simulink model "mppt_fractional_fuzzy_v1"  (R2019a)
settings: Solver=FixedStepAuto  StartTime=0.0  StopTime=3  FixedStep=1e-6  RelTol=1e-3
undefined symbols (not defined in the file): sigbuilder_block, Tpwm
libraries: powerlib x8, fuzblock x1, re_lib x1, eePwmGenerator x1
settings Model: Creator=asus  LastModifiedBy=asus

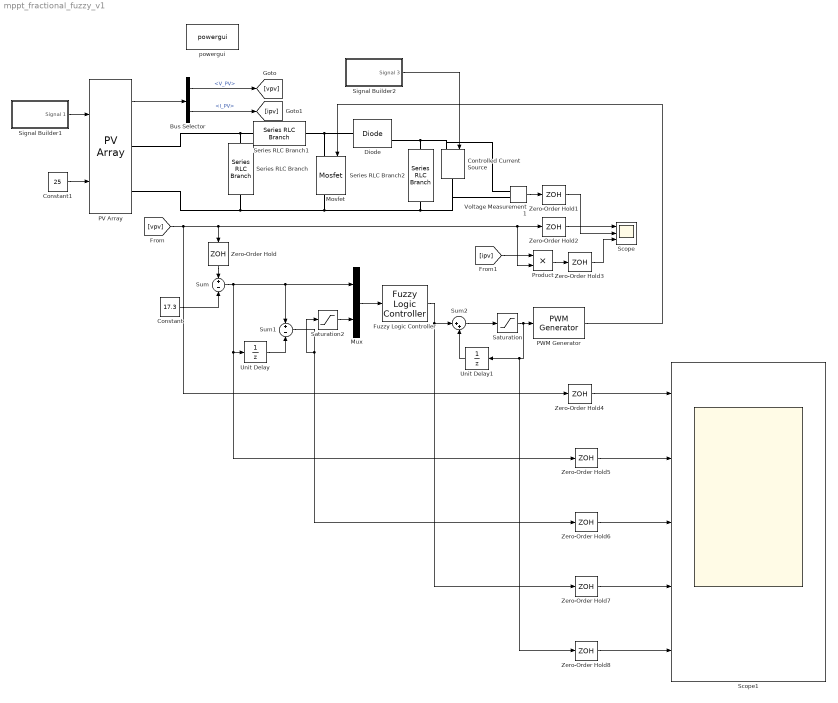
== system mppt_fractional_fuzzy_v1 ==
  Bus Selector : BusSelector  OutputSignals=V_PV,I_PV
  Constant : Constant  Value=17.3
  Constant1 : Constant  Value=25
  Controlled Current Source : powerlib/Electrical Sources/Controlled Current Source  Initialize=on  Source_Type=AC  Amplitude=0  Phase=0  Frequency=0  Measurements=None
      settings: SourceProductName=Simscape Electrical
  Diode : powerlib/Power Electronics/Diode  Ron=0.001  Lon=0  Vf=0.8  IC=0  UseSnubber=0  Rs=500  Cs=250e-9  Measurements=on
      settings: SourceProductName=Simscape Electrical
  Fuzzy Logic Controller : fuzblock/Fuzzy Logic  Controller  FIS=mppt_fractional  OutputSampleNumber=101  DataType=double  FuzzifiedInputs=off  RuleFiringStrengths=off  RuleOutputs=off  AggregatedOutputs=off  SimulateUsing=Interpreted execution  OutOfRangeInputValueMessage=warning  NoRuleFiredMessage=warning  EmptyOutputFuzzySetMessage=warning
  Mosfet : powerlib/Power Electronics/Mosfet  Ron=0.1  Lon=0  Rd=0.01  Vfd=0  IC=0  Rs=1e5  Cs=inf  Measurements=on
      settings: SourceProductName=Simscape Electrical
  Mux : Mux  Inputs=2
  PV Array : re_lib/Solar/PV Array  Npar=1  Nser=1  PlotType=array @ 1000 W/m2 & specified temperatures  S_vec="[ 1000  500  100 ]"  Temp_C_vec="[ 45 25  ]"  ModuleName=Apollo Solar Energy ASEC-120G6M  PlotWhenSelected=off  Pm=120.0969  Ncell=36  Voc=21.6  Isc=7.49  Vm=17.33  Im=6.93  beta_Voc_pc=-0.32991  alpha_Isc_pc=0.021402  beta_Voc=-0.07126  alpha_Isc=0.001603  IL=7.5105  I0=7.9614e-11  nI=0.92533  Rsh=90.7546  Rs=0.24853  BAL=off  Tc=1e-6  Tfilter=5e-5
      settings: SourceProductName=Simscape Electrical
  PWM Generator : eePwmGenerator/PWM Generator  CarrCount=Up  Tper=Tpwm  Ts=1e-6
      settings: SourceProductName=Simscape Electrical
  Product : Product
  Saturation : Saturate  UpperLimit=.98  LowerLimit=.01
  Saturation2 : Saturate  UpperLimit=2.5  LowerLimit=-2.5
  Scope : Scope  NumInputPorts=3
  Scope1 : Scope  NumInputPorts=5
  Series RLC Branch : powerlib/Elements/Series RLC Branch  LConnTagsString=__new0  RConnTagsString=__new0  BranchType=C  Resistance=1  Inductance=1e-3  SetiL0=off  InitialCurrent=0  Capacitance=10e-6  Setx0=off  InitialVoltage=0  Measurements=None
      settings: SourceProductName=Simscape Electrical
  Series RLC Branch1 : powerlib/Elements/Series RLC Branch  LConnTagsString=__new0  RConnTagsString=__new0  BranchType=L  Resistance=1  Inductance=1e-3  SetiL0=off  InitialCurrent=0  Capacitance=10e-6  Setx0=off  InitialVoltage=0  Measurements=None
      settings: SourceProductName=Simscape Electrical
  Series RLC Branch2 : powerlib/Elements/Series RLC Branch  LConnTagsString=__new0  RConnTagsString=__new0  BranchType=C  Resistance=1  Inductance=1e-3  SetiL0=off  InitialCurrent=0  Capacitance=2000e-6  Setx0=off  InitialVoltage=0  Measurements=None
      settings: SourceProductName=Simscape Electrical
  Signal Builder1 : Subsystem  Tag=STV Subsys  LoadFcn=sigbuilder_block('load',[83.5 110.5 550.5 362.5 ]);  StartFcn=sigbuilder_block('start');  StopFcn=sigbuilder_block('stop');  ClipboardFcn=sigbuilder_block('clipboard');  mask(Sigbuilder block){tuvar=[0:10]}
      mask help: Simulink:masks:SigbuilderBlock_MD
      mask init:
      | if ~strcmp(get_param(bdroot(gcbh),'SimulationStatus'),'stopped') tuvar = sigbuilder_block('maskInit'); end
      settings: CopyFcn=sigbuilder_block('copy');  DeleteFcn=sigbuilder_block('delete');  ModelCloseFcn=sigbuilder_block('modelClose');  PreSaveFcn=sigbuilder_block('preSave');  PauseFcn=sigbuilder_block('pause');  ContinueFcn=sigbuilder_block('continue');  NameChangeFcn=sigbuilder_block('namechange');  OpenFcn=sigbuilder_block('open',[83.5 110.5 550.5 362.5 ]);  CloseFcn=sigbuilder_block('close');
      mask Display: plot(0, 0, 100, 100,[2, 2, 32, 32, 2], [68, 8, 8, 68, 68],[32, 2], [38, 38], [32, 19, 2],[53, 60, 44], [32, 17, 17, 2],[16, 16, 31, 31]);txt = getActiveGroup(gcbh);text(2, 100, txt,'verticalAlignment', 'top');
  Signal Builder2 : Subsystem  Tag=STV Subsys  LoadFcn=sigbuilder_block('load',[0 30 960 455.5 ]);  StartFcn=sigbuilder_block('start');  StopFcn=sigbuilder_block('stop');  ClipboardFcn=sigbuilder_block('clipboard');  mask(Sigbuilder block){tuvar=[0:10]}
      mask help: Simulink:masks:SigbuilderBlock_MD
      mask init:
      | if ~strcmp(get_param(bdroot(gcbh),'SimulationStatus'),'stopped') tuvar = sigbuilder_block('maskInit'); end
      settings: CopyFcn=sigbuilder_block('copy');  DeleteFcn=sigbuilder_block('delete');  ModelCloseFcn=sigbuilder_block('modelClose');  PreSaveFcn=sigbuilder_block('preSave');  PauseFcn=sigbuilder_block('pause');  ContinueFcn=sigbuilder_block('continue');  NameChangeFcn=sigbuilder_block('namechange');  OpenFcn=sigbuilder_block('open',[5.5 30 949 418 ]);  CloseFcn=sigbuilder_block('close');
      mask Display: plot(0, 0, 100, 100,[2, 2, 32, 32, 2], [68, 8, 8, 68, 68],[32, 2], [38, 38], [32, 19, 2],[53, 60, 44], [32, 17, 17, 2],[16, 16, 31, 31]);txt = getActiveGroup(gcbh);text(2, 100, txt,'verticalAlignment', 'top');
  Sum : Sum  Inputs=+-
  Sum1 : Sum  Inputs=+-
  Sum2 : Sum  Inputs=|++
  Unit Delay : UnitDelay  SampleTime=-1  HasFrameUpgradeWarning=on
  Unit Delay1 : UnitDelay  SampleTime=-1  HasFrameUpgradeWarning=on
  Voltage Measurement1 : powerlib/Measurements/Voltage Measurement  PhasorSimulation=off  OutputType=Complex  PSBequivalent=0
      settings: SourceProductName=Simscape Electrical
  Zero-Order Hold{,1..8} (9 alike) : ZeroOrderHold  SampleTime=5*Tpwm
  powergui : powerlib/powergui  Priority=1  SimulationMode=Discrete  SampleTime=1e-6  frequency=60  Iterations=50  frequencyindice=0  Pbase=100e6  ErrMax=1e-4  UnitsV=kV  UnitsW=MW  buscounter=0  FunctionMessages=off  echomessages=off  EnableUseOfTLC=off  CurrentSourceSwitches=off  DisableSnubberDevices=off  DisableRonSwitches=off  DisableVfSwitches=off  DisplayEquations=off  AutomaticDiscreteSolvers=off  SolverType=Tustin/Backward Euler (TBE)  Interpol=off  ExternalGateDelay=off  methode=off  Ts=100  x0status=blocks  SPID=on  SwTol=0  HookPort=off  NonlinearTolerance=0  nMaxIteration=15  ContinueOnMaxIteration=off  RestoreLinks=warning  ResistiveCurrentMeasurement=off  Frange=[0:2:500]  Ylog=off  Xlog=on  ShowGrid=off  save=off  variable=ZData  structure=0  ZoomFFT=off  StartTime=0.0  cycles=1  DisplayStyle=1  fundamental=60  FreqAxis=off  MaxFrequency=1000  frequencyindicesteady=1  RmsSteady=1  display=off
      settings: SourceProductName=Simscape Electrical
  wires:
  Signal Builder1/1(Signal 1) -> PV Array/1
  Constant1/1 -> PV Array/2
  Constant/1 -> Sum/2
  Sum2/1 -> Saturation/1
  PWM Generator/1 -> Mosfet/1
  Zero-Order Hold/1 -> Sum/1
  [vpv] -> Zero-Order Hold4/1, Zero-Order Hold/1, Zero-Order Hold2/1, Product/2
  Signal Builder2/1(Signal 3) -> Controlled Current Source/1
  Voltage Measurement1/1 -> Zero-Order Hold1/1
  [ipv] -> Product/1
  Saturation/1 -> Zero-Order Hold8/1, Unit Delay1/1, PWM Generator/1
  PV Array/1 -> Bus Selector/1
  Bus Selector/1 -> [vpv]  "<V_PV>"
  Bus Selector/2 -> [ipv]  "<I_PV>"
  Unit Delay/1 -> Sum1/2
  Sum1/1 -> Saturation2/1, Zero-Order Hold6/1
  Mux/1 -> Fuzzy Logic Controller/1
  Fuzzy Logic Controller/1 -> Zero-Order Hold7/1, Sum2/1
  Unit Delay1/1 -> Sum2/2
  Sum/1 -> Sum1/1, Mux/1, Zero-Order Hold5/1, Unit Delay/1
  Saturation2/1 -> Mux/2
  Zero-Order Hold1/1 -> Scope/2
  Zero-Order Hold2/1 -> Scope/1
  Product/1 -> Zero-Order Hold3/1
  Zero-Order Hold3/1 -> Scope/3
  Zero-Order Hold4/1 -> Scope1/1
  Zero-Order Hold5/1 -> Scope1/2
  Zero-Order Hold6/1 -> Scope1/3
  Zero-Order Hold7/1 -> Scope1/4
  Zero-Order Hold8/1 -> Scope1/5
  connections:
  Series RLC Branch1/LConn1 -- PV Array/RConn1 -- Series RLC Branch/LConn1
  Mosfet/LConn1 -- Diode/LConn1 -- Series RLC Branch1/RConn1
  Mosfet/RConn1 -- Controlled Current Source/RConn1 -- Voltage Measurement1/LConn2 -- Series RLC Branch2/RConn1 -- PV Array/RConn2 -- Series RLC Branch/RConn1
  Diode/RConn1 -- Voltage Measurement1/LConn1 -- Controlled Current Source/LConn1 -- Series RLC Branch2/LConn1

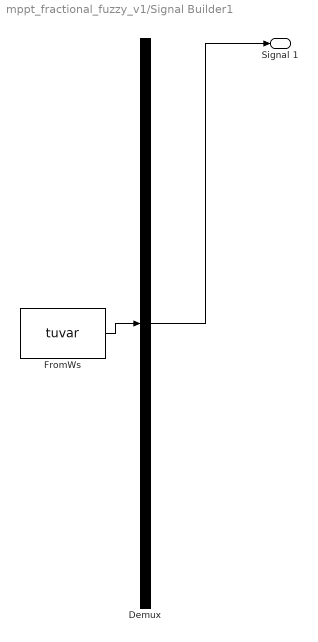
== system mppt_fractional_fuzzy_v1/Signal Builder1 ==
  Demux : Demux  Tag=STV Demux  Outputs=1
  FromWs : FromWorkspace  Tag=STV FromWs  VariableName=tuvar  SampleTime=0
      SigBuilderData=|
      | common.afterFinalStr = 'Extrapolate'
      | common.sampleTime = 0
      | dataSet.timeRange = [0 10]
      | dataSet.name = 'Group 1'
      | sbobj.Groups.Name = 'Group 1'
      | sbobj.Groups.Signals.Name = 'Signal 1'
      | sbobj.Groups.Signals.XData = [0 4.94 4.94 7.96 7.96 10]
      | sbobj.Groups.Signals.YData = [1000 1000 990 990 0 0]
  Signal 1 : Outport  Tag=STV Outport
  wires:
  Demux/1 -> Signal 1/1
  FromWs/1 -> Demux/1

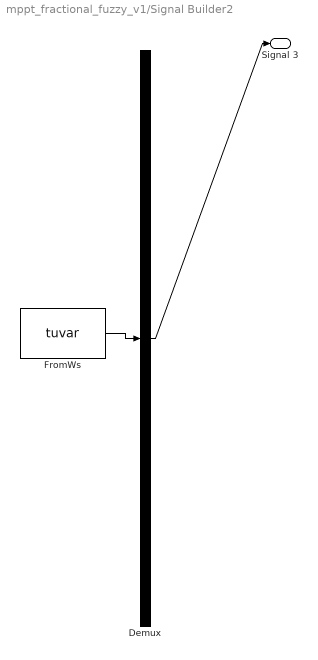
== system mppt_fractional_fuzzy_v1/Signal Builder2 ==
  Demux : Demux  Tag=STV Demux  Outputs=1
  FromWs : FromWorkspace  Tag=STV FromWs  VariableName=tuvar  SampleTime=0
      SigBuilderData=|
      | common.afterFinalStr = 'Extrapolate'
      | common.sampleTime = 0
      | dataSet.timeRange = [0 3]
      | dataSet.name = 'Group 1'
      | sbobj.Groups.Name = 'Group 1'
      | sbobj.Groups.Signals.Name = 'Signal 3'
      | sbobj.Groups.Signals.XData = [0 0.5 0.5 1 1 2 2 3]
      | sbobj.Groups.Signals.YData = [0.995 0.995 6 6 3 3 6 6.00928571429]
      | sbobj.Groups.TimeRange = [0 3]
  Signal 3 : Outport  Tag=STV Outport
  wires:
  FromWs/1 -> Demux/1
  Demux/1 -> Signal 3/1
